simulink model "VSC_3phVoltageSource_VirtImp"  (R2019b)
settings: Solver=ode23tb  StartTime=0.0  StopTime=Tend  RelTol=1e-3
values from neighbouring files (symbols this model uses):
  C_dc = 0.008*(n)    (= 1.6)    [Basic_Model_Works.m]    (also in VSC_GridFroming_Thesis_Script.m; VSC_GridFroming_Thesis_Script_withSynchMach.m)
  C_f = C_f_pu*C1_b    (= 0.0318309886184)    [Basic_Model_Works.m]    (also in VSC_GridFroming_Thesis_Script.m = 0.06; VSC_GridFroming_Thesis_Script_withSynchMach.m)
  f_b = 50    [Basic_Model_Works.m]    (also in VSC_GridFroming_Thesis_Script.m; VSC_GridFroming_Thesis_Script_withSynchMach.m)
  I_b_LV = S_b/(sqrt(3)*V1_rms)    [Basic_Model_Works.m]    (also in VSC_GridFroming_Thesis_Script.m; VSC_GridFroming_Thesis_Script_withSynchMach.m)
  i_ll = -1.15*(S_b/Vdc_n)-i_loss_dc    [Basic_Model_Works.m]    (also in VSC_GridFroming_Thesis_Script.m; VSC_GridFroming_Thesis_Script_withSynchMach.m)
  i_ul = 1.15*(S_b/Vdc_n)+i_loss_dc    [Basic_Model_Works.m]    (also in VSC_GridFroming_Thesis_Script.m; VSC_GridFroming_Thesis_Script_withSynchMach.m)
  k_dc = eta_1/(Vdc_n*m_p)    [Basic_Model_Works.m]    (also in VSC_GridFroming_Thesis_Script.m; VSC_GridFroming_Thesis_Script_withSynchMach.m)
  K_p = (1/Vdc_n)    [Basic_Model_Works.m]    (also in VSC_GridFroming_Thesis_Script.m; VSC_GridFroming_Thesis_Script_withSynchMach.m)
  K_r = 1/R_dc    [Basic_Model_Works.m]    (also in VSC_GridFroming_Thesis_Script.m; VSC_GridFroming_Thesis_Script_withSynchMach.m)
  Kff_i = 1    [Basic_Model_Works.m]    (also in VSC_GridFroming_Thesis_Script.m; VSC_GridFroming_Thesis_Script_withSynchMach.m)
  Kff_v = 1    [Basic_Model_Works.m]    (also in VSC_GridFroming_Thesis_Script.m; VSC_GridFroming_Thesis_Script_withSynchMach.m)
  Ki_i = (1/n)*1.19    (= 0.00595)    [Basic_Model_Works.m]    (also in VSC_GridFroming_Thesis_Script.m; VSC_GridFroming_Thesis_Script_withSynchMach.m)
  Ki_v = (n)*1.16    (= 232)    [Basic_Model_Works.m]    (also in VSC_GridFroming_Thesis_Script.m = 232.2044; VSC_GridFroming_Thesis_Script_withSynchMach.m = 232.2044)
  ki_v_ac = 10    [Basic_Model_Works.m]    (also in VSC_GridFroming_Thesis_Script.m = 0.5; VSC_GridFroming_Thesis_Script_withSynchMach.m)
  Kp_i = 0.73    [Basic_Model_Works.m]    (also in VSC_GridFroming_Thesis_Script.m = 0.738891; VSC_GridFroming_Thesis_Script_withSynchMach.m = 0.738891)
  Kp_v = 0.52    [Basic_Model_Works.m]    (also in VSC_GridFroming_Thesis_Script.m; VSC_GridFroming_Thesis_Script_withSynchMach.m)
  kp_v_ac = 0.05    [Basic_Model_Works.m]    (also in VSC_GridFroming_Thesis_Script.m = 0.001; VSC_GridFroming_Thesis_Script_withSynchMach.m)
  L1_pu = 1*0.0186/m    (= 0.000186)    [Basic_Model_Works.m]    (also in VSC_GridFroming_Thesis_Script.m; VSC_GridFroming_Thesis_Script_withSynchMach.m)
  L2_mh = 0.08    [Basic_Model_Works.m]    (also in VSC_GridFroming_Thesis_Script_withSynchMach.m)
  L_67 = L_lines(5)    [Basic_Model_Works.m]    (also in VSC_GridFroming_Thesis_Script.m; VSC_GridFroming_Thesis_Script_withSynchMach.m)
  L_78 = L_lines(6)    [Basic_Model_Works.m]    (also in VSC_GridFroming_Thesis_Script.m; VSC_GridFroming_Thesis_Script_withSynchMach.m)
  L_f = L_f_pu*L1_b    (= 4.77464829276e-06)    [Basic_Model_Works.m]    (also in VSC_GridFroming_Thesis_Script.m = 1e-06; VSC_GridFroming_Thesis_Script_withSynchMach.m)
  L_v = L_v_pu*L1_b    (= 9.54929658551e-06)    [Basic_Model_Works.m]    (also in VSC_GridFroming_Thesis_Script.m; VSC_GridFroming_Thesis_Script_withSynchMach.m = 9.54929658551e-08)
  m_p = (50*(1.025)-  50*(0.975))/(n*VSC_Pn)    (= 1.25e-08)    [Basic_Model_Works.m]    (also in VSC_GridFroming_Thesis_Script.m = 3.14159265359e-08; VSC_GridFroming_Thesis_Script_withSynchMach.m)
  n = 200    [Basic_Model_Works.m]    (also in VSC_GridFroming_Thesis_Script.m; VSC_GridFroming_Thesis_Script_withSynchMach.m)
  Pn = 210* 1e6    (= 210000000)    [Basic_Model_Works.m]    (also in VSC_GridFroming_Thesis_Script_withSynchMach.m)
  ps = 0.67*Ptot_Load/n_gen    (= 0.5025)    [Basic_Model_Works.m]    (also in VSC_GridFroming_Thesis_Script.m = 0.75; VSC_GridFroming_Thesis_Script_withSynchMach.m = 0.75)
  R1_pu = 1*0.00734/m    (= 7.34e-05)    [Basic_Model_Works.m]    (also in VSC_GridFroming_Thesis_Script.m; VSC_GridFroming_Thesis_Script_withSynchMach.m)
  R2_mh = 0.0027    [Basic_Model_Works.m]    (also in VSC_GridFroming_Thesis_Script_withSynchMach.m)
  R_67 = R_lines(5)    [Basic_Model_Works.m]    (also in VSC_GridFroming_Thesis_Script.m; VSC_GridFroming_Thesis_Script_withSynchMach.m)
  R_78 = R_lines(6)    [Basic_Model_Works.m]    (also in VSC_GridFroming_Thesis_Script.m; VSC_GridFroming_Thesis_Script_withSynchMach.m)
  R_dc = (Vdc_n/(0.05*(S_b)/Vdc_n))    [Basic_Model_Works.m]    (also in VSC_GridFroming_Thesis_Script.m; VSC_GridFroming_Thesis_Script_withSynchMach.m)
  R_f = R_f_pu*Z1_b    (= 5e-05)    [Basic_Model_Works.m]    (also in VSC_GridFroming_Thesis_Script.m = 5e-06; VSC_GridFroming_Thesis_Script_withSynchMach.m)
  R_v = R_v_pu*Z1_b    (= 0.002)    [Basic_Model_Works.m]    (also in VSC_GridFroming_Thesis_Script.m = 0.001; VSC_GridFroming_Thesis_Script_withSynchMach.m = 1e-05)
  S_b = 100*(10^6)    (= 100000000)    [Basic_Model_Works.m]    (also in VSC_GridFroming_Thesis_Script.m; VSC_GridFroming_Thesis_Script_withSynchMach.m)
  T_en = T_conn-0.5    (= 12.5)    [Basic_Model_Works.m]    (also in VSC_GridFroming_Thesis_Script.m = 19.5; VSC_GridFroming_Thesis_Script_withSynchMach.m = 11.5)
  T_load = 20    [VSC_GridFroming_Thesis_Script.m]    (also in VSC_GridFroming_Thesis_Script_withSynchMach.m = 12)
  T_s = 1e-4    (= 0.0001)    [Basic_Model_Works.m]    (also in VSC_GridFroming_Thesis_Script.m; VSC_GridFroming_Thesis_Script_withSynchMach.m)
  tau_dc = 0.05    [Basic_Model_Works.m]    (also in VSC_GridFroming_Thesis_Script.m; VSC_GridFroming_Thesis_Script_withSynchMach.m)
  Tsc_off = 21.15    [Basic_Model_Works.m]    (also in VSC_GridFroming_Thesis_Script_withSynchMach.m = 20.25)
  Tsc_on = 21    [Basic_Model_Works.m]    (also in VSC_GridFroming_Thesis_Script_withSynchMach.m = 20)
  V = 230*(10^3)    (= 230000)    [Basic_Model_Works.m]    (also in VSC_GridFroming_Thesis_Script.m; VSC_GridFroming_Thesis_Script_withSynchMach.m)
  V1_rms = 1000    [Basic_Model_Works.m]    (also in VSC_GridFroming_Thesis_Script.m; VSC_GridFroming_Thesis_Script_withSynchMach.m)
  V2_rms = 13800    [Basic_Model_Works.m]    (also in VSC_GridFroming_Thesis_Script.m; VSC_GridFroming_Thesis_Script_withSynchMach.m)
  V_m = sqrt(2/3)*V1_rms    [Basic_Model_Works.m]    (also in VSC_GridFroming_Thesis_Script.m; VSC_GridFroming_Thesis_Script_withSynchMach.m)
  Vdc_n = 3*V_m    [Basic_Model_Works.m]    (also in VSC_GridFroming_Thesis_Script.m; VSC_GridFroming_Thesis_Script_withSynchMach.m)
  w_c = w_ref/4.95    (= 63.4665182543)    [Basic_Model_Works.m]    (also in VSC_GridFroming_Thesis_Script_withSynchMach.m)
  w_f = 7.5    [Basic_Model_Works.m]    (also in VSC_GridFroming_Thesis_Script.m = 31.4159265359; VSC_GridFroming_Thesis_Script_withSynchMach.m)
  w_ref = 2*pi*f_b    (= 314.159265359)    [Basic_Model_Works.m]    (also in VSC_GridFroming_Thesis_Script.m; VSC_GridFroming_Thesis_Script_withSynchMach.m)
undefined symbols (not defined in the file or in its folder): D1, Delta, i_dc
libraries: powerlib x33, powerlib_meascontrol x10, simulink x1, cstblocks x1
settings Model: Creator=carimjimenez  LastModifiedBy=carimjimenez
settings SolverCC: MaxConsecutiveMinStep=100

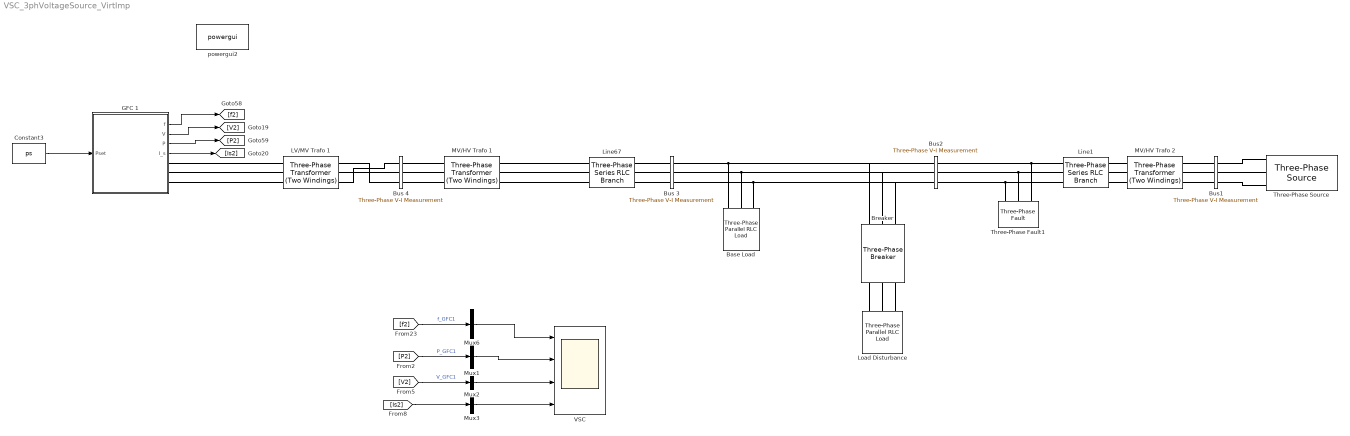
== system VSC_3phVoltageSource_VirtImp ==
  "Base Load " : powerlib/Elements/Three-Phase Parallel RLC Load  LConnTagsString=A|B|C  Configuration=Y (grounded)  NominalVoltage=230e3  Vabc=[1e3 1e3 1e3]  Vabcp=[1e3 1e3 1e3]  NominalFrequency=f_b  UnbalancedPower=off  ActivePower=pl  InductivePower=0  CapacitivePower=0  Pabc=[10e3 9e3 11e3]  QLabc=[100 90 110]  QCabc=[100 90 110]  Pabcp=[10e3 9e3 11e3]  QLabcp=[100 90 110]  QCabcp=[100 90 110]  Measurements=None  LoadType=constant Z
      settings: SourceProductName=Simscape Electrical
  Breaker : powerlib/Elements/Three-Phase Breaker  InitialState=open  SwitchA=on  SwitchB=on  SwitchC=on  SwitchTimes=[T_load]  External=off  BreakerResistance=0.01  SnubberResistance=1e6  SnubberCapacitance=inf  Measurements=None
      settings: SourceProductName=Simscape Electrical
  Bus 3 : powerlib/Measurements/Three-Phase V-I Measurement  VoltageMeasurement=no  SetLabelV=on  LabelV=Vabc_5  Vpu=on  VpuLL=off  CurrentMeasurement=no  SetLabelI=on  LabelI=Iabc_5  Ipu=on  Pbase=S_b  Vbase=V_b  OutputType=Complex  PhasorSimulation=off  PSBequivalent=0
      settings: SourceProductName=Simscape Electrical
  Bus 4 : powerlib/Measurements/Three-Phase V-I Measurement  VoltageMeasurement=no  SetLabelV=on  LabelV=Vabc_8  Vpu=on  VpuLL=off  CurrentMeasurement=no  SetLabelI=on  LabelI=Iabc_8  Ipu=on  Pbase=S_b  Vbase=V_b  OutputType=Complex  PhasorSimulation=off  PSBequivalent=0
      settings: SourceProductName=Simscape Electrical
  Bus1 : powerlib/Measurements/Three-Phase V-I Measurement  VoltageMeasurement=no  SetLabelV=on  LabelV=Vabc_1  Vpu=on  VpuLL=off  CurrentMeasurement=no  SetLabelI=on  LabelI=Iabc_1  Ipu=on  Pbase=S_b  Vbase=V_b  OutputType=Complex  PhasorSimulation=off  PSBequivalent=0
      settings: SourceProductName=Simscape Electrical
  "Bus2 " : powerlib/Measurements/Three-Phase V-I Measurement  VoltageMeasurement=no  SetLabelV=on  LabelV=Vabc_4  Vpu=on  VpuLL=off  CurrentMeasurement=no  SetLabelI=on  LabelI=Iabc_4  Ipu=on  Pbase=S_b  Vbase=V_b  OutputType=Complex  PhasorSimulation=off  PSBequivalent=0
      settings: SourceProductName=Simscape Electrical
  Constant3 : Constant  Value=ps
  GFC 1 : Subsystem
  LV/MV Trafo 1 : powerlib/Elements/Three-Phase Transformer (Two Windings)  Winding1Connection=Yg  Winding2Connection=Yg  CoreType=Three single-phase transformers  SetSaturation=off  Hysteresis=off  DataFile='hysteresis'  SetInitialFlux=off  Measurements=None  UNITS=pu  NominalPower=[S_b f_b ]  Winding1="[ V1_rms R1_pu  L1_pu]"  Winding2=[ V2_rms R1_pu L1_pu]  Rm=Rm_pu  Lm=Lm_pu  L0=0.5  Saturation="[ 0,0  ;  0.005,1.2  ;  1.0,1.4 ]"  InitialFluxes=[ 0.8 , -0.8 , 0.7 ]  BreakLoop=off  DiscreteSolver=Trapezoidal iterative  DataType=off  TransfoNumber=0
      settings: SourceProductName=Simscape Electrical
  Line1 : powerlib/Elements/Three-Phase Series RLC Branch  LConnTagsString=A|B|C  RConnTagsString=A|B|C  BranchType=RL  Resistance=R_78  Inductance=L_78  Capacitance=0  Measurements=None
      settings: SourceProductName=Simscape Electrical
  Line67 : powerlib/Elements/Three-Phase Series RLC Branch  LConnTagsString=A|B|C  RConnTagsString=A|B|C  BranchType=RL  Resistance=R_67  Inductance=L_67  Capacitance=0  Measurements=None
      settings: SourceProductName=Simscape Electrical
  Load Disturbance : powerlib/Elements/Three-Phase Parallel RLC Load  LConnTagsString=A|B|C  Configuration=Y (grounded)  NominalVoltage=230e3  Vabc=[1e3 1e3 1e3]  Vabcp=[1e3 1e3 1e3]  NominalFrequency=f_b  UnbalancedPower=off  ActivePower=load_step  InductivePower=0  CapacitivePower=0  Pabc=[10e3 9e3 11e3]  QLabc=[100 90 110]  QCabc=[100 90 110]  Pabcp=[10e3 9e3 11e3]  QLabcp=[100 90 110]  QCabcp=[100 90 110]  Measurements=None  LoadType=constant Z
      settings: SourceProductName=Simscape Electrical
  MV/HV Trafo 1 : powerlib/Elements/Three-Phase Transformer (Two Windings)  Winding1Connection=Delta (D1)  Winding2Connection=Yg  CoreType=Three single-phase transformers  SetSaturation=off  Hysteresis=off  DataFile='hysteresis'  SetInitialFlux=off  Measurements=None  UNITS=pu  NominalPower=[ Pn f_b ]  Winding1=[V2_rms R2_mh L2_mh]  Winding2=[V R2_mh L2_mh]  Rm=Rm_mh  Lm=Lm_mh  L0=0.5  Saturation="[ 0,0  ;  0.005,1.2  ;  1.0,1.4 ]"  InitialFluxes=[ 0.8 , -0.8 , 0.7 ]  BreakLoop=off  DiscreteSolver=Trapezoidal iterative  DataType=off  TransfoNumber=0
      settings: SourceProductName=Simscape Electrical
  MV/HV Trafo 2 : powerlib/Elements/Three-Phase Transformer (Two Windings)  Winding1Connection=Delta (D1)  Winding2Connection=Yg  CoreType=Three single-phase transformers  SetSaturation=off  Hysteresis=off  DataFile='hysteresis'  SetInitialFlux=off  Measurements=None  UNITS=pu  NominalPower=[ Pn f_b ]  Winding1=[V2_rms R2_mh L2_mh]  Winding2=[V R2_mh L2_mh]  Rm=Rm_mh  Lm=Lm_mh  L0=0.5  Saturation="[ 0,0  ;  0.005,1.2  ;  1.0,1.4 ]"  InitialFluxes=[ 0.8 , -0.8 , 0.7 ]  BreakLoop=off  DiscreteSolver=Trapezoidal iterative  DataType=off  TransfoNumber=0
      settings: SourceProductName=Simscape Electrical
  Mux{1..3,6} (4 alike) : Mux  Inputs=1
  Three-Phase Fault1 : powerlib/Elements/Three-Phase Fault  InitialStates=0  FaultA=on  FaultB=on  FaultC=on  GroundFault=on  SwitchTimes=[Tsc_on Tsc_off]  External=off  SwitchStatus=NaN  FaultResistance=0.001  GroundResistance=0.01  SnubberResistance=1e6  SnubberCapacitance=inf  Measurements=None
      settings: SourceProductName=Simscape Electrical
  Three-Phase Source : powerlib/Electrical Sources/Three-Phase Source  InternalConnection=Yg  VoltagePhases=off  Voltage=V2_rms  PhaseAngle=0  Voltage_phases=[25e3 25e3 25e3]/sqrt(3)  PhaseAngles_phases=[0 -120 +120]  Frequency=f_b  NonIdealSource=off  SpecifyImpedance=off  Resistance=0.8929  Inductance=16.58e-3  ShortCircuitLevel=100e6  BaseVoltage=25e3  XRratio=7  BusType=swing  Pref=10e3  Qref=0  Prefabc=[10e3, 10e3, 10e3]  Qrefabc=[0, 0, 0]  Qmin=-inf  Qmax=inf
      settings: SourceProductName=Simscape Electrical
  VSC : Scope  NumInputPorts=4
  powergui2 : powerlib/powergui  Priority=1  SimulationMode=Discrete  SampleTime=T_s  frequency=50  Iterations=50  frequencyindice=0  Pbase=100e6  ErrMax=0.0001  UnitsV=kV  UnitsW=MW  buscounter=0  FunctionMessages=off  echomessages=off  EnableUseOfTLC=off  CurrentSourceSwitches=off  DisableSnubberDevices=off  DisableRonSwitches=off  DisableVfSwitches=off  DisplayEquations=off  AutomaticDiscreteSolvers=off  SolverType=Tustin/Backward Euler (TBE)  Interpol=off  ExternalGateDelay=off  methode=off  Ts=100  x0status=blocks  SPID=off  SwTol=0  HookPort=off  NonlinearTolerance=1e-4  nMaxIteration=100  ContinueOnMaxIteration=off  RestoreLinks=warning  ResistiveCurrentMeasurement=off  Frange=[0:2:500]  Ylog=off  Xlog=on  ShowGrid=off  save=off  variable=ZData  structure=0  ZoomFFT=off  StartTime=0.0  cycles=1  DisplayStyle=1  fundamental=60  FreqAxis=off  MaxFrequency=1000  frequencyindicesteady=1  RmsSteady=1  display=off
      settings: SourceProductName=Simscape Electrical
  wires:
  [P2] -> Mux1/1  "P_GFC1"
  Mux2/1 -> VSC/3
  Mux3/1 -> VSC/4
  [Is2] -> Mux3/1
  Mux6/1 -> VSC/1
  Mux1/1 -> VSC/2
  [V2] -> Mux2/1  "V_GFC1"
  [f2] -> Mux6/1  "f_GFC1"
  GFC 1/1(f) -> [f2]
  Constant3/1 -> GFC 1/1(Pset)
  GFC 1/4(I_s) -> [Is2]
  GFC 1/2(V) -> [V2]
  GFC 1/3(P) -> [P2]
  connections:
  Line67/RConn1 -- Bus 3/RConn1
  Line67/RConn2 -- Bus 3/RConn2
  Line67/RConn3 -- Bus 3/RConn3
  MV/HV Trafo 1/LConn1 -- Bus 4/RConn1
  Bus 4/RConn2 -- MV/HV Trafo 1/LConn2
  MV/HV Trafo 1/LConn3 -- Bus 4/RConn3
  MV/HV Trafo 1/RConn1 -- Line67/LConn1
  MV/HV Trafo 1/RConn2 -- Line67/LConn2
  MV/HV Trafo 1/RConn3 -- Line67/LConn3
  Bus 3/LConn1 -- "Bus2 "/RConn1 -- Breaker/LConn1 -- "Base Load "/LConn1
  Bus 3/LConn2 -- "Bus2 "/RConn2 -- Breaker/LConn2 -- "Base Load "/LConn2
  Bus 3/LConn3 -- "Bus2 "/RConn3 -- Breaker/LConn3 -- "Base Load "/LConn3
  Breaker/RConn1 -- Load Disturbance/LConn1
  Breaker/RConn2 -- Load Disturbance/LConn2
  Breaker/RConn3 -- Load Disturbance/LConn3
  GFC 1/RConn1 -- LV/MV Trafo 1/LConn3
  Bus 4/LConn1 -- LV/MV Trafo 1/RConn1
  LV/MV Trafo 1/RConn2 -- Bus 4/LConn2
  GFC 1/RConn3 -- LV/MV Trafo 1/LConn1
  GFC 1/RConn2 -- LV/MV Trafo 1/LConn2
  LV/MV Trafo 1/RConn3 -- Bus 4/LConn3
  Line1/RConn3 -- Three-Phase Fault1/LConn3 -- "Bus2 "/LConn3
  Line1/RConn2 -- "Bus2 "/LConn2 -- Three-Phase Fault1/LConn2
  Line1/RConn1 -- Three-Phase Fault1/LConn1 -- "Bus2 "/LConn1
  MV/HV Trafo 2/LConn3 -- Bus1/LConn3
  MV/HV Trafo 2/RConn3 -- Line1/LConn3
  Bus1/RConn2 -- Three-Phase Source/RConn2
  MV/HV Trafo 2/RConn1 -- Line1/LConn1
  MV/HV Trafo 2/LConn1 -- Bus1/LConn1
  Three-Phase Source/RConn3 -- Bus1/RConn3
  MV/HV Trafo 2/RConn2 -- Line1/LConn2
  MV/HV Trafo 2/LConn2 -- Bus1/LConn2
  Three-Phase Source/RConn1 -- Bus1/RConn1

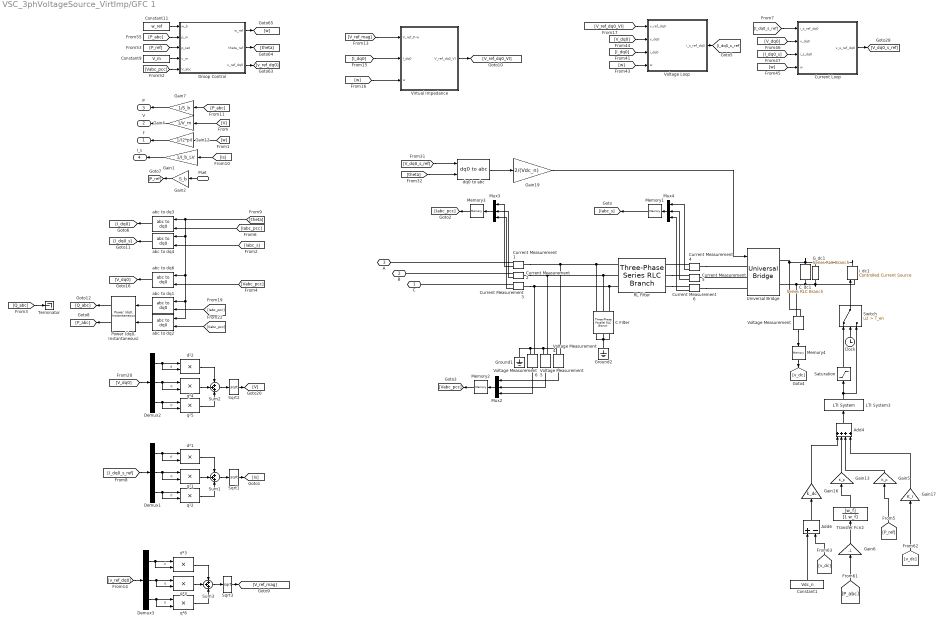
== system VSC_3phVoltageSource_VirtImp/GFC 1 ==
  Pset : Inport
  " Virtual Impedance" : Subsystem
  Add4 : Sum  Inputs=++++
  Add6 : Sum  Inputs=+-
  C Filter : powerlib/Elements/Three-Phase Parallel RLC Branch  LConnTagsString=A|B|C  RConnTagsString=A|B|C  BranchType=C  Resistance=1  Inductance=1e-3  Capacitance=C_f  Measurements=None
      settings: SourceProductName=Simscape Electrical  SourceProductBaseCode=PS
  C_dc1 : powerlib/Elements/Series RLC Branch  LConnTagsString=__new0  RConnTagsString=__new0  BranchType=C  Resistance=1  Inductance=1e-3  SetiL0=off  InitialCurrent=0  Capacitance=C_dc  Setx0=off  InitialVoltage=Vdc_n  Measurements=None
      settings: SourceProductName=Simscape Electrical
  Clock : Clock
  Constant1 : Constant  Value=Vdc_n
  Constant11 : Constant  Value=w_ref
  Constant9 : Constant  Value=V_m
  Current Loop : Subsystem
  Current Measurement{1..6} (6 alike) : powerlib/Measurements/Current Measurement  PhasorSimulation=off  OutputType=Complex  PSBequivalent=0
      settings: SourceProductName=Simscape Electrical
  Demux1 : Demux  Outputs=3
  Demux2 : Demux  Outputs=3
  Demux3 : Demux  Outputs=3
  Droop Control : Subsystem
  G_dc1 : powerlib/Elements/Series RLC Branch  LConnTagsString=__new0  RConnTagsString=__new0  BranchType=R  Resistance=R_dc  Inductance=1e-3  SetiL0=off  InitialCurrent=0  Capacitance=1e-6  Setx0=off  InitialVoltage=0  Measurements=None
      settings: SourceProductName=Simscape Electrical
  Gain1 : Gain  Gain=1/I_b_LV
  Gain12 : Gain  Gain=1/(2*pi)
  Gain13 : Gain  Gain=K_p
  Gain16 : Gain  Gain=k_dc
  Gain17 : Gain  Gain=K_r
  Gain19 : Gain  Gain=2/(Vdc_n)
  Gain2 : Gain  Gain=S_b
  Gain4 : Gain  Gain=1/V_m
  Gain5 : Gain  Gain=K_p
  Gain6 : Gain  Gain=-1
  Gain7 : Gain  Gain=1/S_b
  Ground1 : powerlib/Elements/Ground  LConnTagsString=a
      settings: SourceProductName=Simscape Electrical
  Ground2 : powerlib/Elements/Ground  LConnTagsString=a
      settings: SourceProductName=Simscape Electrical
  LTI System3 : cstblocks/LTI System  sys=tf(1,[tau_dc 1])  IC=[]
  Memory{1..4} (4 alike) : Memory
  Mux2 : Mux  Inputs=3
  Mux3 : Mux  Inputs=3
  Mux4 : Mux  Inputs=3
  "Power (dq0, Instantaneous)" : powerlib_meascontrol/Measurements/Power (dq0, Instantaneous)
      settings: SourceProductName=Simscape Electrical  SourceProductBaseCode=PS
  RL Filter : powerlib/Elements/Three-Phase Series RLC Branch  LConnTagsString=A|B|C  RConnTagsString=A|B|C  BranchType=RL  Resistance=R_f  Inductance=L_f  Capacitance=0  Measurements=None
      settings: SourceProductName=Simscape Electrical
  Saturation : Saturate  UpperLimit=i_ul  LowerLimit=i_ll
  Sqrt1 : Sqrt  SaturateOnIntegerOverflow=on
  Sqrt2 : Sqrt  SaturateOnIntegerOverflow=on
  Sqrt3 : Sqrt  SaturateOnIntegerOverflow=on
  Sum1 : Sum  Inputs=+++  SaturateOnIntegerOverflow=on  InputSameDT=on  OutDataTypeStr=Inherit: Same as first input
  Sum2 : Sum  Inputs=+++  SaturateOnIntegerOverflow=on  InputSameDT=on  OutDataTypeStr=Inherit: Same as first input
  Sum3 : Sum  Inputs=+++  SaturateOnIntegerOverflow=on  InputSameDT=on  OutDataTypeStr=Inherit: Same as first input
  Switch : Switch  Criteria=u2 > Threshold  Threshold=T_en
  Terminator : Terminator
  Transfer Fcn2 : TransferFcn  Numerator=[w_f]  Denominator=[1 w_f]
  Universal Bridge : powerlib/Power Electronics/Universal Bridge  Arms=3  SnubberResistance=1e5  SnubberCapacitance=inf  Device=Average-model based VSC  Ron=1e-3  Lon=0  ForwardVoltages="[  0  0  ]"  ForwardVoltage=0  GTOparameters=[ 10e-6 , 20e-6 ]  IGBTparameters=[ 1e-6 , 2e-6 ]  Measurements=None  Measurements_2=None  converterType=Rectifier
      settings: SourceProductName=Simscape Electrical
  Voltage Loop : Subsystem
  Voltage Measurement{,4..6} (4 alike) : powerlib/Measurements/Voltage Measurement  PhasorSimulation=off  OutputType=Complex  PSBequivalent=0
      settings: SourceProductName=Simscape Electrical
  abc to dq{1..4,6} (5 alike) : powerlib_meascontrol/Transformations/abc to dq0  Alignment=90 degrees behind phase A axis
      settings: SourceProductName=Simscape Electrical
  dq0 to abc : powerlib_meascontrol/Transformations/dq0 to abc  Alignment=90 degrees behind phase A axis
      settings: SourceProductName=Simscape Electrical
  d²1 : Product  SaturateOnIntegerOverflow=on  RndMeth=Zero  InputSameDT=on  OutDataTypeStr=Inherit: Same as first input
  d²2 : Product  SaturateOnIntegerOverflow=on  RndMeth=Zero  InputSameDT=on  OutDataTypeStr=Inherit: Same as first input
  d²3 : Product  SaturateOnIntegerOverflow=on  RndMeth=Zero  InputSameDT=on  OutDataTypeStr=Inherit: Same as first input
  i_dc1 : powerlib/Electrical Sources/Controlled Current Source  Initialize=off  Source_Type=DC  Amplitude=i_dc  Phase=0  Frequency=0  Measurements=None
      settings: SourceProductName=Simscape Electrical
  q²{1..6} (6 alike) : Product  SaturateOnIntegerOverflow=on  RndMeth=Zero  InputSameDT=on  OutDataTypeStr=Inherit: Same as first input
  C : PMIOPort  Side=Right
  B : PMIOPort  Port=2  Side=Right
  A : PMIOPort  Port=3  Side=Right
  f : Outport  VectorParamsAs1DForOutWhenUnconnected=off
  V : Outport  Port=2  VectorParamsAs1DForOutWhenUnconnected=off
  P : Outport  Port=3  VectorParamsAs1DForOutWhenUnconnected=off
  I_s : Outport  Port=4  VectorParamsAs1DForOutWhenUnconnected=off
  wires:
  Gain7/1 -> P/1
  [P_abc] -> Gain7/1
  Current Measurement6/1 -> Mux4/3
  Current Measurement5/1 -> Mux4/2
  Current Measurement4/1 -> Mux4/1
  Current Measurement3/1 -> Mux3/3
  Current Measurement2/1 -> Mux3/2
  Current Measurement1/1 -> Mux3/1
  Voltage Measurement4/1 -> Mux2/1
  Voltage Measurement5/1 -> Mux2/2
  Voltage Measurement6/1 -> Mux2/3
  [V] -> Gain4/1
  Gain2/1 -> [P_ref]
  Pset/1 -> Gain2/1
  Gain12/1 -> f/1
  [w] -> Gain12/1
  Mux2/1 -> Memory2/1
  Mux3/1 -> Memory3/1
  abc to dq1/1 -> "Power (dq0, Instantaneous)"/2
  abc to dq2/1 -> "Power (dq0, Instantaneous)"/1
  [Vabc_pcc] -> abc to dq2/1
  "Power (dq0, Instantaneous)"/2 -> [Q_abc]
  "Power (dq0, Instantaneous)"/1 -> [P_abc]
  [Iabc_pcc] -> abc to dq1/1
  Gain4/1 -> V/1
  [Iabc_pcc] -> abc to dq3/1
  [Iabc_s] -> abc to dq4/1
  [Vabc_pcc] -> abc to dq6/1
  [theta] -> abc to dq2/2, abc to dq1/2, abc to dq6/2, abc to dq4/2, abc to dq3/2
  abc to dq3/1 -> [I_dq0]
  abc to dq4/1 -> [I_dq0_s]
  abc to dq6/1 -> [V_dq0]
  [theta] -> dq0 to abc/2
  q²4/1 -> Sum2/2
  [V_dq0] -> Demux2/1
  q²5/1 -> Sum2/3
  Sum2/1 -> Sqrt2/1
  Demux2/3 -> q²5/1, q²5/2  "0"
  d²2/1 -> Sum2/1
  Demux2/2 -> q²4/1, q²4/2  "q"
  Demux2/1 -> d²2/1, d²2/2  "d"
  Sqrt2/1 -> [V]
  Mux4/1 -> Memory1/1
  Memory2/1 -> [Vabc_pcc]
  Memory3/1 -> [Iabc_pcc]
  Memory1/1 -> [Iabc_s]
  dq0 to abc/1 -> Gain19/1
  [w] -> Current Loop/4(w)
  [V_ref_dq0_VI] -> Voltage Loop/1(v_ref_dq0)
  [I_dq0] -> Voltage Loop/3(i_dq0)
  [V_dq0] -> Current Loop/2(v_dq0)
  [I_dq0_s] -> Current Loop/3(i_s_dq0)
  Current Loop/1(v_s_ref_dq0) -> [V_dq0_s_ref]
  [w] -> Voltage Loop/4(w)
  [V_dq0] -> Voltage Loop/2(v_dq0)
  Switch/1 -> i_dc1/1
  Gain19/1 -> Universal Bridge/1
  [V_dq0_s_ref] -> dq0 to abc/1
  Constant11/1 -> Droop Control/1(w_b)
  Droop Control/3(v_ref_dq0) -> [v_ref_dq0]
  [P_abc] -> Droop Control/2(p_m)
  Constant9/1 -> Droop Control/4(v_m)
  [Vabc_pcc] -> Droop Control/5(V_abc)
  Droop Control/2(theta_ref) -> [theta]
  Droop Control/1(w_ref) -> [w]
  [P_ref] -> Droop Control/3(p_set)
  Gain16/1 -> Add4/1
  Gain6/1 -> Transfer Fcn2/1
  [P_ref] -> Gain5/1
  Memory4/1 -> [v_dc]
  Add4/1 -> LTI System3/1
  [v_dc] -> Gain17/1
  Gain13/1 -> Add4/2
  Add6/1 -> Gain16/1
  Voltage Measurement/1 -> Memory4/1
  Clock/1 -> Switch/2
  [P_abc] -> Gain6/1
  Constant1/1 -> Add6/1
  Gain5/1 -> Add4/3
  Gain17/1 -> Add4/4
  LTI System3/1 -> Switch/3, Saturation/1
  Transfer Fcn2/1 -> Gain13/1
  Saturation/1 -> Switch/1
  [v_dc] -> Add6/2
  [Q_abc] -> Terminator/1
  Voltage Loop/1(i_s_ref_dq0) -> [I_dq0_s_ref]
  [I_dq0_s_ref] -> Current Loop/1(i_s_ref_dq0)
  q²2/1 -> Sum1/3
  Demux1/2 -> q²1/1, q²1/2  "q"
  [I_dq0_s_ref] -> Demux1/1
  Demux1/1 -> d²1/1, d²1/2  "d"
  Sum1/1 -> Sqrt1/1
  Demux1/3 -> q²2/1, q²2/2  "0"
  Sqrt1/1 -> [Is]
  d²1/1 -> Sum1/1
  q²1/1 -> Sum1/2
  [Is] -> Gain1/1
  Gain1/1 -> I_s/1
  [v_ref_dq0] -> Demux3/1
  Demux3/2 -> q²3/1, q²3/2  "q"
  Demux3/1 -> d²3/1, d²3/2  "d"
  q²3/1 -> Sum3/2
  q²6/1 -> Sum3/3
  Sum3/1 -> Sqrt3/1
  Demux3/3 -> q²6/1, q²6/2  "0"
  d²3/1 -> Sum3/1
  Sqrt3/1 -> [V_ref_mag]
  [V_ref_mag] -> " Virtual Impedance"/1("V_ref_P-w ")
  [I_dq0] -> " Virtual Impedance"/2(I_dq0)
  [w] -> " Virtual Impedance"/3(w)
  " Virtual Impedance"/1(V_ref_dq0_VI) -> [V_ref_dq0_VI]
  connections:
  Current Measurement2/LConn1 -- C Filter/LConn2 -- RL Filter/RConn2 -- Voltage Measurement5/LConn1
  Voltage Measurement6/LConn1 -- RL Filter/RConn3 -- C Filter/LConn3 -- Current Measurement3/LConn1
  Universal Bridge/RConn1 -- i_dc1/RConn1 -- G_dc1/LConn1 -- C_dc1/LConn1 -- Voltage Measurement/LConn1
  Voltage Measurement6/LConn2 -- Voltage Measurement5/LConn2 -- Voltage Measurement4/LConn2 -- Ground1/LConn1
  Current Measurement3/RConn1 -- C/RConn1
  Current Measurement2/RConn1 -- B/RConn1
  Current Measurement1/RConn1 -- A/RConn1
  Current Measurement6/LConn1 -- Universal Bridge/LConn3
  Current Measurement5/LConn1 -- Universal Bridge/LConn2
  Current Measurement4/LConn1 -- Universal Bridge/LConn1
  Universal Bridge/RConn2 -- i_dc1/LConn1 -- G_dc1/RConn1 -- C_dc1/RConn1 -- Voltage Measurement/LConn2
  RL Filter/RConn1 -- C Filter/LConn1 -- Voltage Measurement4/LConn1 -- Current Measurement1/LConn1
  C Filter/RConn1 -- Ground2/LConn1 -- C Filter/RConn2 -- C Filter/RConn3
  Current Measurement4/RConn1 -- RL Filter/LConn1
  RL Filter/LConn2 -- Current Measurement5/RConn1
  RL Filter/LConn3 -- Current Measurement6/RConn1

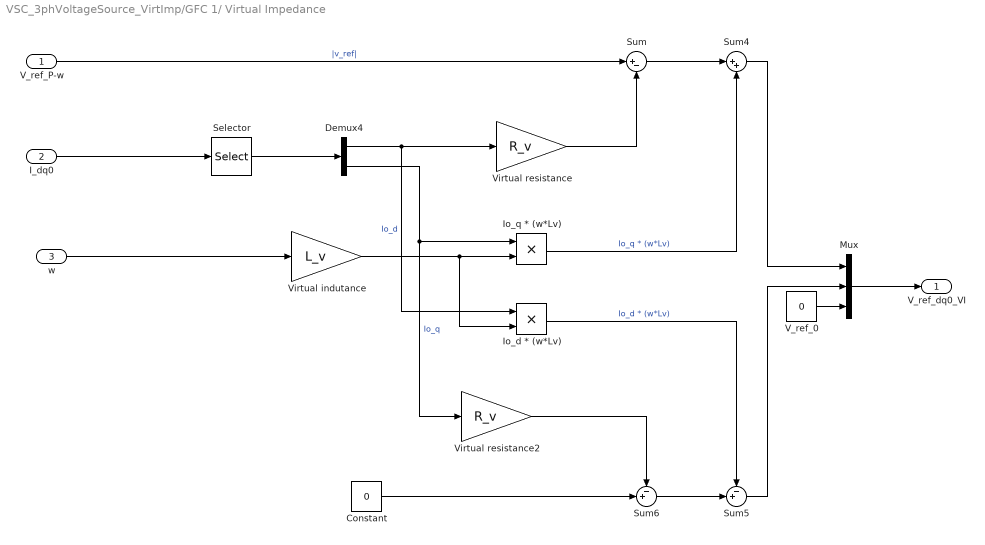
== system VSC_3phVoltageSource_VirtImp/GFC 1/ Virtual Impedance ==
  "V_ref_P-w " : Inport
  I_dq0 : Inport  Port=2
  w : Inport  Port=3
  Constant : Constant  Value=0
  Demux4 : Demux  Outputs=2
  "Io_d * (w*Lv) " : Product  RndMeth=Zero
  "Io_q * (w*Lv) " : Product  RndMeth=Zero
  Mux : Mux  Inputs=3
  Selector : Selector  InputPortWidth=3  IndexOptions=Index vector (dialog)  Indices=[1 2]  OutputSizes=1
  Sum : Sum  Inputs=|+-
  Sum4 : Sum  Inputs=|++
  Sum5 : Sum  Inputs=-+|
  Sum6 : Sum  Inputs=-+|
  V_ref_0 : Constant  Value=0
  Virtual indutance : Gain  Gain=L_v
  Virtual resistance : Gain  Gain=R_v
  "Virtual resistance2 " : Gain  Gain=R_v
  V_ref_dq0_VI : Outport
  wires:
  "Io_d * (w*Lv) "/1 -> Sum5/1  "Io_d * (w*Lv)"
  Sum4/1 -> Mux/1
  Virtual indutance/1 -> "Io_q * (w*Lv) "/2, "Io_d * (w*Lv) "/2
  Sum/1 -> Sum4/1
  I_dq0/1 -> Selector/1
  w/1 -> Virtual indutance/1
  Virtual resistance/1 -> Sum/2
  "Virtual resistance2 "/1 -> Sum6/1
  Sum5/1 -> Mux/2
  Selector/1 -> Demux4/1
  Sum6/1 -> Sum5/2
  V_ref_0/1 -> Mux/3
  Demux4/1 -> "Io_d * (w*Lv) "/1, Virtual resistance/1  "Io_d"
  "V_ref_P-w "/1 -> Sum/1  "|v_ref|"
  Constant/1 -> Sum6/2
  "Io_q * (w*Lv) "/1 -> Sum4/2  "Io_q * (w*Lv)"
  Demux4/2 -> "Virtual resistance2 "/1, "Io_q * (w*Lv) "/1  "Io_q"
  Mux/1 -> V_ref_dq0_VI/1

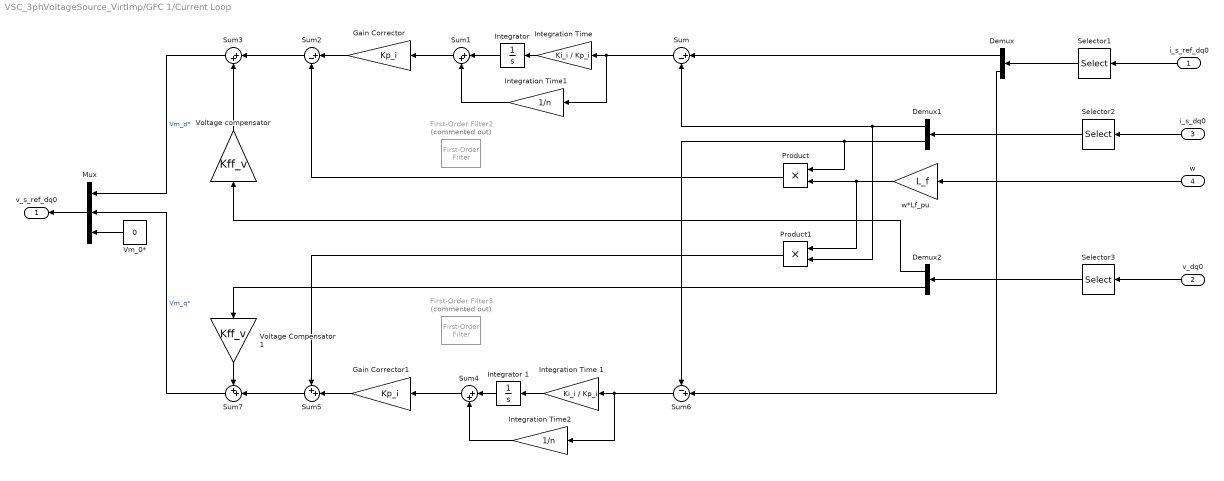
== system VSC_3phVoltageSource_VirtImp/GFC 1/Current Loop ==
  i_s_ref_dq0 : Inport
  v_dq0 : Inport  Port=2
  i_s_dq0 : Inport  Port=3
  w : Inport  Port=4
  Demux : Demux  Outputs=2
  Demux1 : Demux  Outputs=2
  Demux2 : Demux  Outputs=2
  First-Order Filter2 : powerlib_meascontrol/Filters/First-Order Filter  Commented=on  FilterType=Lowpass  Tc=25e-3  Ts=0  Initialize=on  Vac_Init=[0, 0, 50]  Vdc_Init=1  PlotResponse=off  FreqRange="[0,  200,  1]"
      settings: SourceProductName=Simscape Electrical
  First-Order Filter3 : powerlib_meascontrol/Filters/First-Order Filter  Commented=on  FilterType=Lowpass  Tc=25e-3  Ts=0  Initialize=on  Vac_Init=[0, 0, 50]  Vdc_Init=0  PlotResponse=off  FreqRange="[0,  200,  1]"
      settings: SourceProductName=Simscape Electrical
  Gain Corrector : Gain  Gain=Kp_i
  Gain Corrector1 : Gain  Gain=Kp_i
  Integration Time : Gain  Gain=Ki_i / Kp_i
  Integration Time 1 : Gain  Gain=Ki_i / Kp_i
  Integration Time1 : Gain  Gain=1/n
  Integration Time2 : Gain  Gain=1/n
  Integrator : Integrator  InitialCondition=0.0001
  Integrator 1 : Integrator
  Mux : Mux  Inputs=3
  Product : Product  RndMeth=Zero
  Product1 : Product  RndMeth=Zero
  Selector1 : Selector  InputPortWidth=3  IndexOptions=Index vector (dialog)  Indices=[1 2]  OutputSizes=1
  Selector2 : Selector  InputPortWidth=3  IndexOptions=Index vector (dialog)  Indices=[1 2]  OutputSizes=1
  Selector3 : Selector  InputPortWidth=3  IndexOptions=Index vector (dialog)  Indices=[1 2]  OutputSizes=1
  Sum : Sum  Inputs=|+-
  Sum1 : Sum  Inputs=|++
  Sum2 : Sum  Inputs=|+-
  Sum3 : Sum  Inputs=|++
  Sum4 : Sum  Inputs=|++
  Sum5 : Sum  Inputs=++|
  Sum6 : Sum  Inputs=-+|
  Sum7 : Sum  Inputs=++|
  Vm_0* : Constant  Value=0
  Voltage Compensator 1 : Gain  Gain=Kff_v
  Voltage compensator : Gain  Gain=Kff_v
  w*Lf_pu : Gain  Gain=L_f
  v_s_ref_dq0 : Outport  VectorParamsAs1DForOutWhenUnconnected=off
  wires:
  Sum/1 -> Integration Time/1, Integration Time1/1
  Integration Time 1/1 -> Integrator 1/1
  Integration Time/1 -> Integrator/1
  Sum5/1 -> Sum7/2
  Sum6/1 -> Integration Time 1/1, Integration Time2/1
  Demux/1 -> Sum/1
  Sum3/1 -> Mux/1  "Vm_d*"
  Sum7/1 -> Mux/2  "Vm_q*"
  Demux2/2 -> Voltage Compensator 1/1
  Voltage Compensator 1/1 -> Sum7/1
  Product/1 -> Sum2/2
  w*Lf_pu/1 -> Product1/1, Product/2
  i_s_ref_dq0/1 -> Selector1/1
  v_dq0/1 -> Selector3/1
  Integrator 1/1 -> Sum4/1
  Voltage compensator/1 -> Sum3/2
  Sum1/1 -> Gain Corrector/1
  Sum2/1 -> Sum3/1
  Sum4/1 -> Gain Corrector1/1
  Demux/2 -> Sum6/2
  Selector1/1 -> Demux/1
  Gain Corrector/1 -> Sum2/1
  w/1 -> w*Lf_pu/1
  Mux/1 -> v_s_ref_dq0/1
  Selector2/1 -> Demux1/1
  i_s_dq0/1 -> Selector2/1
  Selector3/1 -> Demux2/1
  Demux1/2 -> Product/1, Sum6/1
  Vm_0*/1 -> Mux/3
  Integrator/1 -> Sum1/1
  Demux1/1 -> Product1/2, Sum/2
  Demux2/1 -> Voltage compensator/1
  Product1/1 -> Sum5/1
  Gain Corrector1/1 -> Sum5/2
  Integration Time1/1 -> Sum1/2
  Integration Time2/1 -> Sum4/2

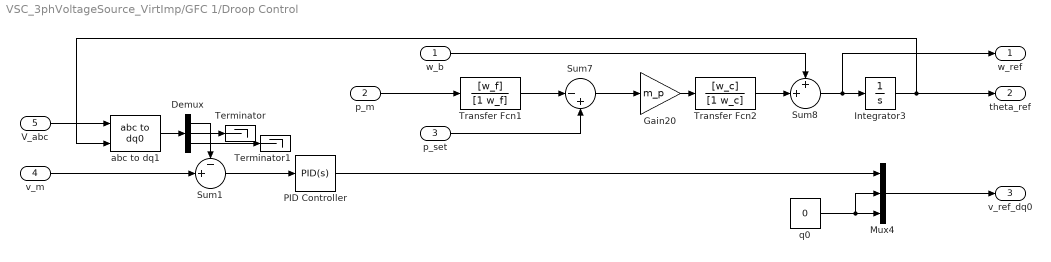
== system VSC_3phVoltageSource_VirtImp/GFC 1/Droop Control ==
  w_b : Inport
  p_m : Inport  Port=2
  p_set : Inport  Port=3
  v_m : Inport  Port=4
  V_abc : Inport  Port=5
  Demux : Demux  Outputs=3
  Gain20 : Gain  Gain=m_p
  Integrator3 : Integrator
  Mux4 : Mux  Inputs=3
  PID Controller : simulink/Continuous/PID Controller  Controller=PID  Form=Parallel  TimeDomain=Continuous-time  SampleTime=-1  IntegratorMethod=Forward Euler  FilterMethod=Forward Euler  ControllerParametersSource=internal  P=kp_v_ac  I=ki_v_ac  D=0  UseFilter=on  N=100  TunerSelectOption=Transfer Function Based (PID Tuner App)  InitialConditionSource=internal  InitialConditionForIntegrator=0  InitialConditionForFilter=0  DifferentiatorICPrevScaledInput=0  ExternalReset=none  TrackingMode=off  Kt=1  LimitOutput=off  UpperSaturationLimit=inf  LowerSaturationLimit=-inf  LinearizeAsGain=on  AntiWindupMode=none  Kb=1  POutMin=[]  POutMax=[]  IOutMin=[]  IOutMax=[]  DOutMin=[]  DOutMax=[]  NOutMin=[]  NOutMax=[]  SumOutMin=[]  SumOutMax=[]  SaturationOutMin=[]  SaturationOutMax=[]  PParamMin=[]  PParamMax=[]  IParamMin=[]  IParamMax=[]  DParamMin=[]  DParamMax=[]  NParamMin=[]  NParamMax=[]  KbParamMin=[]  KbParamMax=[]  KtParamMin=[]  KtParamMax=[]  KbOutMin=[]  KbOutMax=[]  KtOutMin=[]  KtOutMax=[]  IntegratorOutMin=[]  IntegratorOutMax=[]  FilterOutMin=[]  FilterOutMax=[]  SumI1OutMin=[]  SumI1OutMax=[]  SumI2OutMin=[]  SumI2OutMax=[]  SumI3OutMin=[]  SumI3OutMax=[]  SumI4OutMin=[]  SumI4OutMax=[]  SumDOutMin=[]  SumDOutMax=[]  DifferentiatorOutMin=[]  DifferentiatorOutMax=[]  FilterDiffOutCoefMin=[]  FilterDiffOutCoefMax=[]  ReciprocalOutMin=[]  ReciprocalOutMax=[]  SumDenOutMin=[]  SumDenOutMax=[]  SumNumOutMin=[]  SumNumOutMax=[]  DivideOutMin=[]  DivideOutMax=[]  IntegratorContinuousStateAttributes=''  IntegratorStateMustResolveToSignalObject=off  IntegratorRTWStateStorageClass=Auto  FilterContinuousStateAttributes=''  FilterStateMustResolveToSignalObject=off  FilterRTWStateStorageClass=Auto  ParallelPVariant=InternalParameters  IdealPVariant=Disabled  IVariant=InternalParameters  DVariant=InternalParameters  IntegratorVariant=Continuous  SatVariant=Disabled  AWVariant=Passthrough  PCopyVariant=Disabled  TRVariant=Disabled  FdbkBlocksVariant=Forward  IdealPFdbkVariant=Disabled  SatFdbkVariant=Disabled  DerivativeFilterVariant=ContFilter  NVariant=InternalParameters  NCopyVariant=Disabled  FilterICVariant=InternalICsFilter  IntegratorICVariant=InternalICs  ExternalResetVariant=Disabled  TRSumVariant=Passthrough  SumFdbkVariant=Disabled  SumVariant=Sum_PID
  Sum1 : Sum  Inputs=-+|
  Sum7 : Sum  Inputs=|-+
  Sum8 : Sum  Inputs=++|
  Terminator : Terminator
  Terminator1 : Terminator
  Transfer Fcn1 : TransferFcn  Numerator=[w_f]  Denominator=[1 w_f]
  Transfer Fcn2 : TransferFcn  Numerator=[w_c]  Denominator=[1 w_c]
  abc to dq1 : powerlib_meascontrol/Transformations/abc to dq0  Alignment=90 degrees behind phase A axis
      settings: SourceProductName=Simscape Electrical
  q0 : Constant  Value=0
  w_ref : Outport  VectorParamsAs1DForOutWhenUnconnected=off
  theta_ref : Outport  Port=2  VectorParamsAs1DForOutWhenUnconnected=off
  v_ref_dq0 : Outport  Port=3  VectorParamsAs1DForOutWhenUnconnected=off
  wires:
  Demux/1 -> Sum1/1
  abc to dq1/1 -> Demux/1
  Mux4/1 -> v_ref_dq0/1
  q0/1 -> Mux4/3, Mux4/2
  Sum8/1 -> Integrator3/1, w_ref/1
  p_set/1 -> Sum7/2
  w_b/1 -> Sum8/1
  V_abc/1 -> abc to dq1/1
  Sum1/1 -> PID Controller/1
  v_m/1 -> Sum1/2
  Integrator3/1 -> abc to dq1/2, theta_ref/1
  PID Controller/1 -> Mux4/1
  Demux/2 -> Terminator/1
  Demux/3 -> Terminator1/1
  p_m/1 -> Transfer Fcn1/1
  Sum7/1 -> Gain20/1
  Transfer Fcn1/1 -> Sum7/1
  Gain20/1 -> Transfer Fcn2/1
  Transfer Fcn2/1 -> Sum8/2

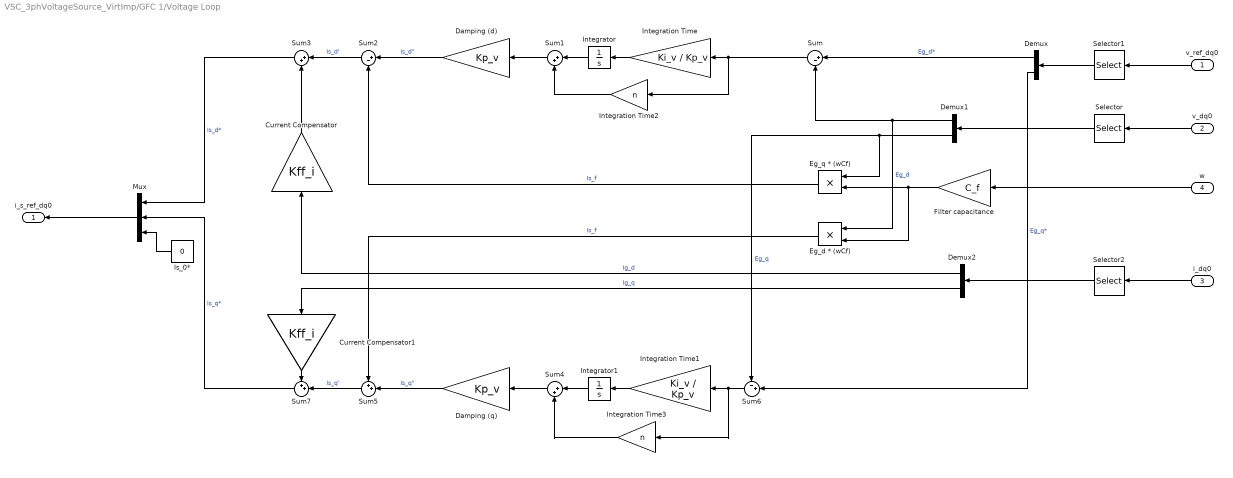
== system VSC_3phVoltageSource_VirtImp/GFC 1/Voltage Loop ==
  v_ref_dq0 : Inport
  v_dq0 : Inport  Port=2
  i_dq0 : Inport  Port=3
  w : Inport  Port=4
  Current Compensator : Gain  Gain=Kff_i
  Current Compensator1 : Gain  Gain=Kff_i
  Damping (d) : Gain  Gain=Kp_v
  Damping (q) : Gain  Gain=Kp_v
  Demux : Demux  Outputs=2
  Demux1 : Demux  Outputs=2
  Demux2 : Demux  Outputs=2
  Eg_d * (wCf) : Product  RndMeth=Zero
  "Eg_q * (wCf) " : Product  RndMeth=Zero
  Filter capacitance : Gain  Gain=C_f
  Integration Time : Gain  Gain=Ki_v / Kp_v
  Integration Time1 : Gain  Gain=Ki_v / Kp_v
  Integration Time2 : Gain  Gain=n
  Integration Time3 : Gain  Gain=n
  Integrator : Integrator
  Integrator1 : Integrator
  Is_0* : Constant  Value=0
  Mux : Mux  Inputs=3
  Selector : Selector  InputPortWidth=3  IndexOptions=Index vector (dialog)  Indices=[1 2]  OutputSizes=1
  Selector1 : Selector  InputPortWidth=3  IndexOptions=Index vector (dialog)  Indices=[1 2]  OutputSizes=1
  Selector2 : Selector  InputPortWidth=3  IndexOptions=Index vector (dialog)  Indices=[1 2]  OutputSizes=1
  Sum : Sum  Inputs=|+-
  Sum1 : Sum  Inputs=|++
  Sum2 : Sum  Inputs=|+-
  Sum3 : Sum  Inputs=|++
  Sum4 : Sum  Inputs=|++
  Sum5 : Sum  Inputs=++|
  Sum6 : Sum  Inputs=-+|
  Sum7 : Sum  Inputs=++|
  i_s_ref_dq0 : Outport  VectorParamsAs1DForOutWhenUnconnected=off
  wires:
  Is_0*/1 -> Mux/3
  w/1 -> Filter capacitance/1
  Integration Time1/1 -> Integrator1/1
  Integrator1/1 -> Sum4/1
  Demux/2 -> Sum6/2  "Eg_q*"
  v_ref_dq0/1 -> Selector1/1
  Eg_d * (wCf)/1 -> Sum5/1  "Is_f"
  Sum7/1 -> Mux/2  "Is_q*"
  Demux2/2 -> Current Compensator1/1  "Ig_q"
  Demux/1 -> Sum/1  "Eg_d*"
  Sum6/1 -> Integration Time3/1, Integration Time1/1
  Demux2/1 -> Current Compensator/1  "Ig_d"
  Sum2/1 -> Sum3/1  "Is_d'"
  Current Compensator/1 -> Sum3/2
  Demux1/1 -> Eg_d * (wCf)/1, Sum/2  "Eg_d"
  Current Compensator1/1 -> Sum7/1
  "Eg_q * (wCf) "/1 -> Sum2/2  "Is_f"
  Demux1/2 -> "Eg_q * (wCf) "/1, Sum6/1  "Eg_q"
  Filter capacitance/1 -> "Eg_q * (wCf) "/2, Eg_d * (wCf)/2
  Damping (d)/1 -> Sum2/1  "Is_d\""
  i_dq0/1 -> Selector2/1
  Sum5/1 -> Sum7/2  "Is_q'"
  Sum1/1 -> Damping (d)/1
  Integrator/1 -> Sum1/1
  Integration Time/1 -> Integrator/1
  Sum4/1 -> Damping (q)/1
  Sum3/1 -> Mux/1  "Is_d*"
  v_dq0/1 -> Selector/1
  Damping (q)/1 -> Sum5/2  "Is_q\""
  Selector/1 -> Demux1/1
  Selector1/1 -> Demux/1
  Selector2/1 -> Demux2/1
  Mux/1 -> i_s_ref_dq0/1
  Sum/1 -> Integration Time/1, Integration Time2/1
  Integration Time2/1 -> Sum1/2
  Integration Time3/1 -> Sum4/2
